simulink model "Hell_ix_System_Architecture"  (R2022b)
settings: Solver=VariableStepAuto  StartTime=0.0  StopTime=10.0  RelTol=1e-3
(part 1 of 2)
settings Model: Creator=Daniel Sotelo  LastModifiedBy=Daniel Sotelo

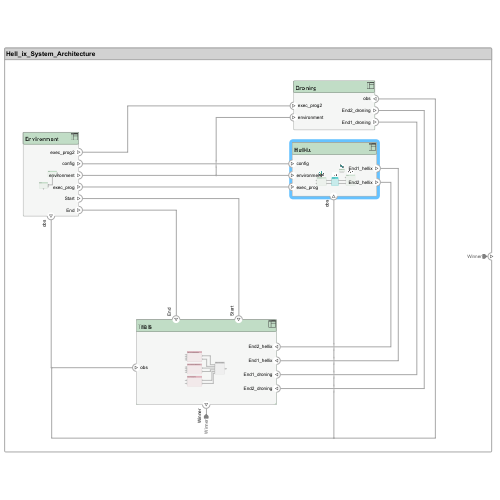
[thumbnail: Simulink's stored preview of the top-level diagram]
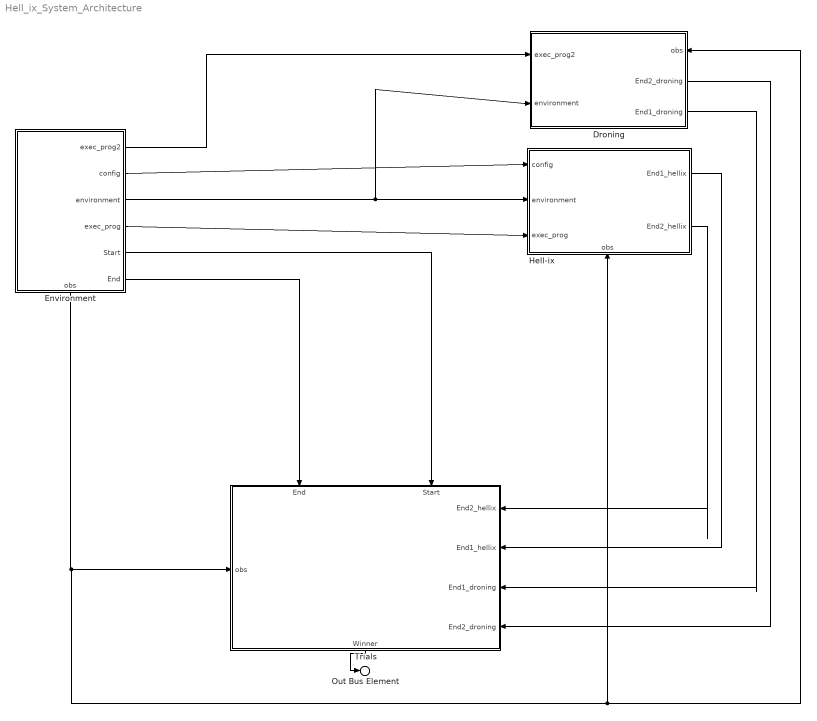
== system Hell_ix_System_Architecture ==
  Droning : Subsystem
      settings: PortSchema="{\"entries\":[{\"content\":{\"headerSize\":26,\"margin\":15,\"minimumSpacing\":25,\"sides\":[{\"content\":{\"connectorIds\":[\"In2\",\"In1\"]},\"type\":\"ConnectorPlacement.EquallySpacedRectSide\",\"uuid\":\"e97e1fd1-9f1b-43cc-bf15-a23fe97b9f57\"},{\"content\":{\"connectorIds\":[\"In3\",\"Out2\",\"Out1\"],\"side\":\"RIGHT\"},\"type\":\"ConnectorPlacement.EquallySpacedRectSide\",\"uuid\":\"b384b9c5-fcee-4054-b020-18cc4d409726\"},{\"content\":{\"connectorIds\":[],\"side\":\"TOP\"},\"type\":\"ConnectorPlacement.EquallySpacedRectSide\",\"uuid\":\"0ff74274-cc13-4bc9-ab97-befa0144ddb0\"}]},\"type\":\"ConnectorPlacement.EquallySpacedConnector\",\"uuid\":\"32a64cae-dc0e-47e5-be72-f6041fa7e3a1\"}],\"packageUris\":[\"http://schema.mathworks.com/mf0/Connector/R2020b\"],\"version\":\"1.0\"}"
  Environment : Subsystem
      settings: PortSchema="{\"entries\":[{\"content\":{\"headerSize\":26,\"margin\":15,\"minimumSpacing\":25,\"sides\":[{\"content\":{\"connectorIds\":[]},\"type\":\"ConnectorPlacement.EquallySpacedRectSide\",\"uuid\":\"e97e1fd1-9f1b-43cc-bf15-a23fe97b9f57\"},{\"content\":{\"connectorIds\":[\"Out3\",\"Out2\",\"Out1\",\"Out4\",\"Out5\",\"Out6\"],\"side\":\"RIGHT\"},\"type\":\"ConnectorPlacement.EquallySpacedRectSide\",\"uuid\":\"b384b9c5-fcee-4054-b020-18cc4d409726\"},{\"content\":{\"connectorIds\":[],\"side\":\"TOP\"},\"type\":\"ConnectorPlacement.EquallySpacedRectSide\",\"uuid\":\"0ff74274-cc13-4bc9-ab97-befa0144ddb0\"},{\"content\":{\"connectorIds\":[\"Out7\"],\"side\":\"BOTTOM\"},\"type\":\"ConnectorPlacement.EquallySpacedRectSide\",\"uuid\":\"34d21596-7255-4b53-b653-035a383f4a5b\"}]},\"type\":\"ConnectorPlacement.EquallySpacedConnector\",\"uuid\":\"32a64cae-dc0e-47e5-be72-f6041fa7e3a1\"}],\"packageUris\":[\"http://schema.mathworks.com/mf0/Connector/R2020b\"],\"version\":\"1.0\"}"
  Hell-ix : Subsystem
      settings: PortSchema="{\"entries\":[{\"content\":{\"headerSize\":26,\"margin\":15,\"minimumSpacing\":25,\"sides\":[{\"content\":{\"connectorIds\":[\"In1\",\"In2\",\"In3\"]},\"type\":\"ConnectorPlacement.EquallySpacedRectSide\",\"uuid\":\"e97e1fd1-9f1b-43cc-bf15-a23fe97b9f57\"},{\"content\":{\"connectorIds\":[\"Out2\",\"Out1\"],\"side\":\"RIGHT\"},\"type\":\"ConnectorPlacement.EquallySpacedRectSide\",\"uuid\":\"b384b9c5-fcee-4054-b020-18cc4d409726\"},{\"content\":{\"connectorIds\":[],\"side\":\"TOP\"},\"type\":\"ConnectorPlacement.EquallySpacedRectSide\",\"uuid\":\"0ff74274-cc13-4bc9-ab97-befa0144ddb0\"},{\"content\":{\"connectorIds\":[\"In4\"],\"side\":\"BOTTOM\"},\"type\":\"ConnectorPlacement.EquallySpacedRectSide\",\"uuid\":\"8630347b-1320-4b67-a4d6-78d4ff5f81b4\"}]},\"type\":\"ConnectorPlacement.EquallySpacedConnector\",\"uuid\":\"32a64cae-dc0e-47e5-be72-f6041fa7e3a1\"}],\"packageUris\":[\"http://schema.mathworks.com/mf0/Connector/R2020b\"],\"version\":\"1.0\"}"
  Trials : Subsystem
      settings: PortSchema="{\"entries\":[{\"content\":{\"headerSize\":26,\"margin\":15,\"minimumSpacing\":25,\"sides\":[{\"content\":{\"connectorIds\":[\"In7\"]},\"type\":\"ConnectorPlacement.EquallySpacedRectSide\",\"uuid\":\"e97e1fd1-9f1b-43cc-bf15-a23fe97b9f57\"},{\"content\":{\"connectorIds\":[\"In5\",\"In6\",\"In3\",\"In4\"],\"side\":\"RIGHT\"},\"type\":\"ConnectorPlacement.EquallySpacedRectSide\",\"uuid\":\"b384b9c5-fcee-4054-b020-18cc4d409726\"},{\"content\":{\"connectorIds\":[\"In2\",\"In1\"],\"side\":\"TOP\"},\"type\":\"ConnectorPlacement.EquallySpacedRectSide\",\"uuid\":\"0ff74274-cc13-4bc9-ab97-befa0144ddb0\"},{\"content\":{\"connectorIds\":[\"Out1\"],\"side\":\"BOTTOM\"},\"type\":\"ConnectorPlacement.EquallySpacedRectSide\",\"uuid\":\"9cacfc43-c38e-4776-99af-1c6d2f7a9023\"}]},\"type\":\"ConnectorPlacement.EquallySpacedConnector\",\"uuid\":\"32a64cae-dc0e-47e5-be72-f6041fa7e3a1\"}],\"packageUris\":[\"http://schema.mathworks.com/mf0/Connector/R2020b\"],\"version\":\"1.0\"}"
  Out Bus Element : Outport  PortName=Winner
  wires:
  Environment/4(exec_prog) -> Hell-ix/3(exec_prog)
  Environment/7(obs) -> Trials/7(obs), Hell-ix/4(obs), Droning/3(obs)
  Environment/6(End) -> Trials/2(End)
  Environment/3(exec_prog2) -> Droning/2(exec_prog2)
  Environment/5(Start) -> Trials/1(Start)
  Environment/1(environment) -> Droning/1(environment), Hell-ix/2(environment)
  Droning/1(End1_droning) -> Trials/3(End1_droning)
  Droning/2(End2_droning) -> Trials/4(End2_droning)
  Hell-ix/1(End2_hellix) -> Trials/5(End2_hellix)
  Hell-ix/2(End1_hellix) -> Trials/6(End1_hellix)
  Trials/1(Winner) -> Out Bus Element/1
  Environment/2(config) -> Hell-ix/1(config)

== system Hell_ix_System_Architecture/Droning ==
  Bus Element In3 : Inport  PortName=environment
  Bus Element In1 : Inport  Port=2  PortName=exec_prog2
  Bus Element In2 : Inport  Port=3  PortName=obs
  Bus Element Out1 : Outport  PortName=End1_droning
  Bus Element Out2 : Outport  Port=2  PortName=End2_droning

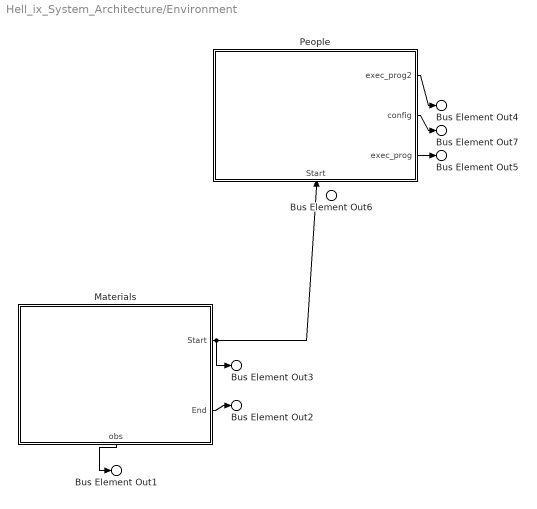
== system Hell_ix_System_Architecture/Environment ==
  Materials : Subsystem
      settings: PortSchema="{\"entries\":[{\"content\":{\"headerSize\":26,\"margin\":15,\"minimumSpacing\":25,\"sides\":[{\"content\":{\"connectorIds\":[]},\"type\":\"ConnectorPlacement.EquallySpacedRectSide\",\"uuid\":\"e97e1fd1-9f1b-43cc-bf15-a23fe97b9f57\"},{\"content\":{\"connectorIds\":[\"Out1\",\"Out3\"],\"side\":\"RIGHT\"},\"type\":\"ConnectorPlacement.EquallySpacedRectSide\",\"uuid\":\"b384b9c5-fcee-4054-b020-18cc4d409726\"},{\"content\":{\"connectorIds\":[],\"side\":\"TOP\"},\"type\":\"ConnectorPlacement.EquallySpacedRectSide\",\"uuid\":\"0ff74274-cc13-4bc9-ab97-befa0144ddb0\"},{\"content\":{\"connectorIds\":[\"Out2\"],\"side\":\"BOTTOM\"},\"type\":\"ConnectorPlacement.EquallySpacedRectSide\",\"uuid\":\"156d3aac-f76d-47d1-8807-e77bc3f5e7ef\"}]},\"type\":\"ConnectorPlacement.EquallySpacedConnector\",\"uuid\":\"32a64cae-dc0e-47e5-be72-f6041fa7e3a1\"}],\"packageUris\":[\"http://schema.mathworks.com/mf0/Connector/R2020b\"],\"version\":\"1.0\"}"
  People : Subsystem
      settings: PortSchema="{\"entries\":[{\"content\":{\"headerSize\":26,\"margin\":15,\"minimumSpacing\":25,\"sides\":[{\"content\":{\"connectorIds\":[]},\"type\":\"ConnectorPlacement.EquallySpacedRectSide\",\"uuid\":\"e97e1fd1-9f1b-43cc-bf15-a23fe97b9f57\"},{\"content\":{\"connectorIds\":[\"Out3\",\"Out2\",\"Out1\"],\"side\":\"RIGHT\"},\"type\":\"ConnectorPlacement.EquallySpacedRectSide\",\"uuid\":\"b384b9c5-fcee-4054-b020-18cc4d409726\"},{\"content\":{\"connectorIds\":[],\"side\":\"TOP\"},\"type\":\"ConnectorPlacement.EquallySpacedRectSide\",\"uuid\":\"0ff74274-cc13-4bc9-ab97-befa0144ddb0\"},{\"content\":{\"connectorIds\":[\"In1\"],\"side\":\"BOTTOM\"},\"type\":\"ConnectorPlacement.EquallySpacedRectSide\",\"uuid\":\"a378ab0b-ffdd-4b76-9379-7a6c14cd9027\"}]},\"type\":\"ConnectorPlacement.EquallySpacedConnector\",\"uuid\":\"32a64cae-dc0e-47e5-be72-f6041fa7e3a1\"}],\"packageUris\":[\"http://schema.mathworks.com/mf0/Connector/R2020b\"],\"version\":\"1.0\"}"
  Bus Element Out6 : Outport  PortName=environment
  Bus Element Out7 : Outport  Port=2  PortName=config
  Bus Element Out4 : Outport  Port=3  PortName=exec_prog2
  Bus Element Out5 : Outport  Port=4  PortName=exec_prog
  Bus Element Out3 : Outport  Port=5  PortName=Start
  Bus Element Out2 : Outport  Port=6  PortName=End
  Bus Element Out1 : Outport  Port=7  PortName=obs
  wires:
  Materials/2(obs) -> Bus Element Out1/1
  Materials/3(End) -> Bus Element Out2/1
  Materials/1(Start) -> People/1(Start), Bus Element Out3/1
  People/3(exec_prog2) -> Bus Element Out4/1
  People/1(exec_prog) -> Bus Element Out5/1
  People/2(config) -> Bus Element Out7/1

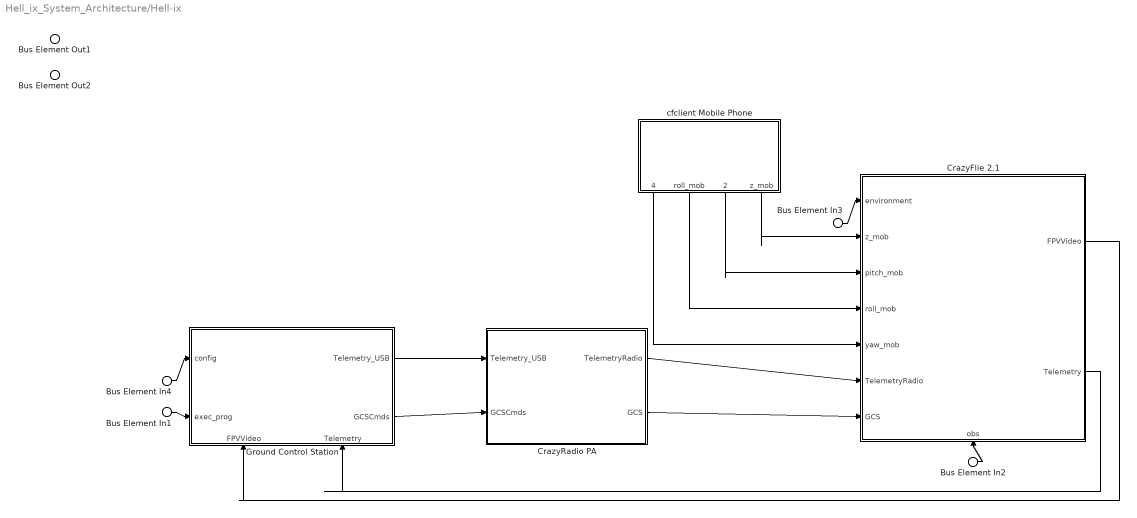
== system Hell_ix_System_Architecture/Hell-ix ==
  Bus Element In4 : Inport  PortName=config
  Bus Element In3 : Inport  Port=2  PortName=environment
  Bus Element In1 : Inport  Port=3  PortName=exec_prog
  Bus Element In2 : Inport  Port=4  PortName=obs
  CrazyFlie 2.1 : Subsystem
      settings: PortSchema="{\"entries\":[{\"content\":{\"headerSize\":26,\"margin\":15,\"minimumSpacing\":25,\"sides\":[{\"content\":{\"connectorIds\":[\"In2\",\"In4\",\"In5\",\"In6\",\"In7\",\"In3\",\"In8\"]},\"type\":\"ConnectorPlacement.EquallySpacedRectSide\",\"uuid\":\"e97e1fd1-9f1b-43cc-bf15-a23fe97b9f57\"},{\"content\":{\"connectorIds\":[\"Out2\",\"Out1\"],\"side\":\"RIGHT\"},\"type\":\"ConnectorPlacement.EquallySpacedRectSide\",\"uuid\":\"b384b9c5-fcee-4054-b020-18cc4d409726\"},{\"content\":{\"connectorIds\":[],\"side\":\"TOP\"},\"type\":\"ConnectorPlacement.EquallySpacedRectSide\",\"uuid\":\"0ff74274-cc13-4bc9-ab97-befa0144ddb0\"},{\"content\":{\"connectorIds\":[\"In1\"],\"side\":\"BOTTOM\"},\"type\":\"ConnectorPlacement.EquallySpacedRectSide\",\"uuid\":\"e7cf066c-a9d0-4f44-9f2b-ff8a675b3a93\"}]},\"type\":\"ConnectorPlacement.EquallySpacedConnector\",\"uuid\":\"32a64cae-dc0e-47e5-be72-f6041fa7e3a1\"}],\"packageUris\":[\"http://schema.mathworks.com/mf0/Connector/R2020b\"],\"version\":\"1.0\"}"
  CrazyRadio PA : Subsystem
      settings: PortSchema="{\"entries\":[{\"content\":{\"headerSize\":26,\"margin\":15,\"minimumSpacing\":25,\"sides\":[{\"content\":{\"connectorIds\":[\"In1\",\"In2\"]},\"type\":\"ConnectorPlacement.EquallySpacedRectSide\",\"uuid\":\"e97e1fd1-9f1b-43cc-bf15-a23fe97b9f57\"},{\"content\":{\"connectorIds\":[\"Out1\",\"Out2\"],\"side\":\"RIGHT\"},\"type\":\"ConnectorPlacement.EquallySpacedRectSide\",\"uuid\":\"b384b9c5-fcee-4054-b020-18cc4d409726\"},{\"content\":{\"connectorIds\":[],\"side\":\"TOP\"},\"type\":\"ConnectorPlacement.EquallySpacedRectSide\",\"uuid\":\"0ff74274-cc13-4bc9-ab97-befa0144ddb0\"}]},\"type\":\"ConnectorPlacement.EquallySpacedConnector\",\"uuid\":\"32a64cae-dc0e-47e5-be72-f6041fa7e3a1\"}],\"packageUris\":[\"http://schema.mathworks.com/mf0/Connector/R2020b\"],\"version\":\"1.0\"}"
  Ground Control Station : Subsystem
      settings: PortSchema="{\"entries\":[{\"content\":{\"headerSize\":26,\"margin\":15,\"minimumSpacing\":25,\"sides\":[{\"content\":{\"connectorIds\":[\"In1\",\"In2\"]},\"type\":\"ConnectorPlacement.EquallySpacedRectSide\",\"uuid\":\"e97e1fd1-9f1b-43cc-bf15-a23fe97b9f57\"},{\"content\":{\"connectorIds\":[\"Out1\",\"Out2\"],\"side\":\"RIGHT\"},\"type\":\"ConnectorPlacement.EquallySpacedRectSide\",\"uuid\":\"b384b9c5-fcee-4054-b020-18cc4d409726\"},{\"content\":{\"connectorIds\":[],\"side\":\"TOP\"},\"type\":\"ConnectorPlacement.EquallySpacedRectSide\",\"uuid\":\"0ff74274-cc13-4bc9-ab97-befa0144ddb0\"},{\"content\":{\"connectorIds\":[\"In3\",\"In4\"],\"side\":\"BOTTOM\"},\"type\":\"ConnectorPlacement.EquallySpacedRectSide\",\"uuid\":\"d255ce1e-bd8c-464a-9c5c-901bed1a1a29\"}]},\"type\":\"ConnectorPlacement.EquallySpacedConnector\",\"uuid\":\"32a64cae-dc0e-47e5-be72-f6041fa7e3a1\"}],\"packageUris\":[\"http://schema.mathworks.com/mf0/Connector/R2020b\"],\"version\":\"1.0\"}"
  cfclient Mobile Phone : Subsystem
      settings: PortSchema="{\"entries\":[{\"content\":{\"headerSize\":26,\"margin\":15,\"minimumSpacing\":25,\"sides\":[{\"content\":{\"connectorIds\":[]},\"type\":\"ConnectorPlacement.EquallySpacedRectSide\",\"uuid\":\"e97e1fd1-9f1b-43cc-bf15-a23fe97b9f57\"},{\"content\":{\"connectorIds\":[],\"side\":\"RIGHT\"},\"type\":\"ConnectorPlacement.EquallySpacedRectSide\",\"uuid\":\"b384b9c5-fcee-4054-b020-18cc4d409726\"},{\"content\":{\"connectorIds\":[],\"side\":\"TOP\"},\"type\":\"ConnectorPlacement.EquallySpacedRectSide\",\"uuid\":\"0ff74274-cc13-4bc9-ab97-befa0144ddb0\"},{\"content\":{\"connectorIds\":[\"Out4\",\"Out3\",\"Out2\",\"Out1\"],\"side\":\"BOTTOM\"},\"type\":\"ConnectorPlacement.EquallySpacedRectSide\",\"uuid\":\"6bcd37d7-be34-4491-8512-8c3ebf2e5fa9\"}]},\"type\":\"ConnectorPlacement.EquallySpacedConnector\",\"uuid\":\"32a64cae-dc0e-47e5-be72-f6041fa7e3a1\"}],\"packageUris\":[\"http://schema.mathworks.com/mf0/Connector/R2020b\"],\"version\":\"1.0\"}"
  Bus Element Out1 : Outport  PortName=End2_hellix
  Bus Element Out2 : Outport  Port=2  PortName=End1_hellix
  wires:
  Ground Control Station/1(Telemetry_USB) -> CrazyRadio PA/1(Telemetry_USB)
  Ground Control Station/2(GCSCmds) -> CrazyRadio PA/2(GCSCmds)
  CrazyRadio PA/2(GCS) -> CrazyFlie 2.1/8(GCS)
  CrazyRadio PA/1(TelemetryRadio) -> CrazyFlie 2.1/3(TelemetryRadio)
  Bus Element In1/1 -> Ground Control Station/2(exec_prog)
  Bus Element In4/1 -> Ground Control Station/1(config)
  Bus Element In3/1 -> CrazyFlie 2.1/2(environment)
  CrazyFlie 2.1/2(FPVVideo) -> Ground Control Station/3(FPVVideo)
  cfclient Mobile Phone/1(z_mob) -> CrazyFlie 2.1/4(z_mob)
  cfclient Mobile Phone/2(pitch_mob) -> CrazyFlie 2.1/5(pitch_mob)
  cfclient Mobile Phone/3(roll_mob) -> CrazyFlie 2.1/6(roll_mob)
  cfclient Mobile Phone/4(yaw_mob) -> CrazyFlie 2.1/7(yaw_mob)
  Bus Element In2/1 -> CrazyFlie 2.1/1(obs)
  CrazyFlie 2.1/1(Telemetry) -> Ground Control Station/4(Telemetry)

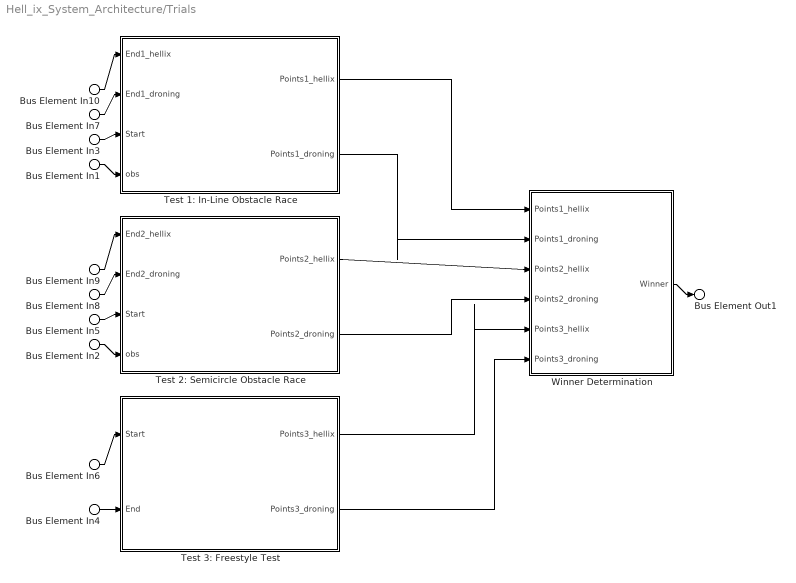
== system Hell_ix_System_Architecture/Trials ==
  Bus Element In3 : Inport  PortName=Start
  Bus Element In5 : Inport  PortName=Start
  Bus Element In6 : Inport  PortName=Start
  Bus Element In4 : Inport  Port=2  PortName=End
  Bus Element In7 : Inport  Port=3  PortName=End1_droning
  Bus Element In8 : Inport  Port=4  PortName=End2_droning
  Bus Element In9 : Inport  Port=5  PortName=End2_hellix
  Bus Element In10 : Inport  Port=6  PortName=End1_hellix
  Bus Element In1 : Inport  Port=7  PortName=obs
  Bus Element In2 : Inport  Port=7  PortName=obs
  Test 1: In-Line Obstacle Race : Subsystem
      settings: PortSchema="{\"entries\":[{\"content\":{\"headerSize\":26,\"margin\":15,\"minimumSpacing\":25,\"sides\":[{\"content\":{\"connectorIds\":[\"In1\",\"In2\",\"In3\",\"In4\"]},\"type\":\"ConnectorPlacement.EquallySpacedRectSide\",\"uuid\":\"e97e1fd1-9f1b-43cc-bf15-a23fe97b9f57\"},{\"content\":{\"connectorIds\":[\"Out1\",\"Out2\"],\"side\":\"RIGHT\"},\"type\":\"ConnectorPlacement.EquallySpacedRectSide\",\"uuid\":\"b384b9c5-fcee-4054-b020-18cc4d409726\"},{\"content\":{\"connectorIds\":[],\"side\":\"TOP\"},\"type\":\"ConnectorPlacement.EquallySpacedRectSide\",\"uuid\":\"0ff74274-cc13-4bc9-ab97-befa0144ddb0\"}]},\"type\":\"ConnectorPlacement.EquallySpacedConnector\",\"uuid\":\"32a64cae-dc0e-47e5-be72-f6041fa7e3a1\"}],\"packageUris\":[\"http://schema.mathworks.com/mf0/Connector/R2020b\"],\"version\":\"1.0\"}"
  Test 2: Semicircle Obstacle Race : Subsystem
      settings: PortSchema="{\"entries\":[{\"content\":{\"headerSize\":26,\"margin\":15,\"minimumSpacing\":25,\"sides\":[{\"content\":{\"connectorIds\":[\"In1\",\"In2\",\"In3\",\"In4\"]},\"type\":\"ConnectorPlacement.EquallySpacedRectSide\",\"uuid\":\"e97e1fd1-9f1b-43cc-bf15-a23fe97b9f57\"},{\"content\":{\"connectorIds\":[\"Out1\",\"Out2\"],\"side\":\"RIGHT\"},\"type\":\"ConnectorPlacement.EquallySpacedRectSide\",\"uuid\":\"b384b9c5-fcee-4054-b020-18cc4d409726\"},{\"content\":{\"connectorIds\":[],\"side\":\"TOP\"},\"type\":\"ConnectorPlacement.EquallySpacedRectSide\",\"uuid\":\"0ff74274-cc13-4bc9-ab97-befa0144ddb0\"}]},\"type\":\"ConnectorPlacement.EquallySpacedConnector\",\"uuid\":\"32a64cae-dc0e-47e5-be72-f6041fa7e3a1\"}],\"packageUris\":[\"http://schema.mathworks.com/mf0/Connector/R2020b\"],\"version\":\"1.0\"}"
  Test 3: Freestyle Test : Subsystem
      settings: PortSchema="{\"entries\":[{\"content\":{\"headerSize\":26,\"margin\":15,\"minimumSpacing\":25,\"sides\":[{\"content\":{\"connectorIds\":[\"In1\",\"In2\"]},\"type\":\"ConnectorPlacement.EquallySpacedRectSide\",\"uuid\":\"e97e1fd1-9f1b-43cc-bf15-a23fe97b9f57\"},{\"content\":{\"connectorIds\":[\"Out1\",\"Out2\"],\"side\":\"RIGHT\"},\"type\":\"ConnectorPlacement.EquallySpacedRectSide\",\"uuid\":\"b384b9c5-fcee-4054-b020-18cc4d409726\"},{\"content\":{\"connectorIds\":[],\"side\":\"TOP\"},\"type\":\"ConnectorPlacement.EquallySpacedRectSide\",\"uuid\":\"0ff74274-cc13-4bc9-ab97-befa0144ddb0\"}]},\"type\":\"ConnectorPlacement.EquallySpacedConnector\",\"uuid\":\"32a64cae-dc0e-47e5-be72-f6041fa7e3a1\"}],\"packageUris\":[\"http://schema.mathworks.com/mf0/Connector/R2020b\"],\"version\":\"1.0\"}"
  Winner Determination : Subsystem
      settings: PortSchema="{\"entries\":[{\"content\":{\"headerSize\":26,\"margin\":15,\"minimumSpacing\":25,\"sides\":[{\"content\":{\"connectorIds\":[\"In2\",\"In1\",\"In3\",\"In4\",\"In6\",\"In5\"]},\"type\":\"ConnectorPlacement.EquallySpacedRectSide\",\"uuid\":\"e97e1fd1-9f1b-43cc-bf15-a23fe97b9f57\"},{\"content\":{\"connectorIds\":[\"Out1\"],\"side\":\"RIGHT\"},\"type\":\"ConnectorPlacement.EquallySpacedRectSide\",\"uuid\":\"b384b9c5-fcee-4054-b020-18cc4d409726\"},{\"content\":{\"connectorIds\":[],\"side\":\"TOP\"},\"type\":\"ConnectorPlacement.EquallySpacedRectSide\",\"uuid\":\"0ff74274-cc13-4bc9-ab97-befa0144ddb0\"}]},\"type\":\"ConnectorPlacement.EquallySpacedConnector\",\"uuid\":\"32a64cae-dc0e-47e5-be72-f6041fa7e3a1\"}],\"packageUris\":[\"http://schema.mathworks.com/mf0/Connector/R2020b\"],\"version\":\"1.0\"}"
  Bus Element Out1 : Outport  PortName=Winner
  wires:
  Bus Element In1/1 -> Test 1: In-Line Obstacle Race/4(obs)
  Bus Element In2/1 -> Test 2: Semicircle Obstacle Race/4(obs)
  Bus Element In3/1 -> Test 1: In-Line Obstacle Race/3(Start)
  Bus Element In5/1 -> Test 2: Semicircle Obstacle Race/3(Start)
  Bus Element In6/1 -> Test 3: Freestyle Test/1(Start)
  Bus Element In4/1 -> Test 3: Freestyle Test/2(End)
  Bus Element In7/1 -> Test 1: In-Line Obstacle Race/2(End1_droning)
  Bus Element In10/1 -> Test 1: In-Line Obstacle Race/1(End1_hellix)
  Bus Element In8/1 -> Test 2: Semicircle Obstacle Race/2(End2_droning)
  Bus Element In9/1 -> Test 2: Semicircle Obstacle Race/1(End2_hellix)
  Test 1: In-Line Obstacle Race/1(Points1_hellix) -> Winner Determination/2(Points1_hellix)
  Test 1: In-Line Obstacle Race/2(Points1_droning) -> Winner Determination/1(Points1_droning)
  Test 2: Semicircle Obstacle Race/1(Points2_hellix) -> Winner Determination/3(Points2_hellix)
  Test 2: Semicircle Obstacle Race/2(Points2_droning) -> Winner Determination/4(Points2_droning)
  Test 3: Freestyle Test/1(Points3_hellix) -> Winner Determination/6(Points3_hellix)
  Test 3: Freestyle Test/2(Points3_droning) -> Winner Determination/5(Points3_droning)
  Winner Determination/1(Winner) -> Bus Element Out1/1

== system Hell_ix_System_Architecture/Environment/Materials ==
  Chronometer : Subsystem
      settings: PortSchema="{\"entries\":[{\"content\":{\"headerSize\":26,\"margin\":15,\"minimumSpacing\":25,\"sides\":[{\"content\":{\"connectorIds\":[\"In1\"]},\"type\":\"ConnectorPlacement.EquallySpacedRectSide\",\"uuid\":\"e97e1fd1-9f1b-43cc-bf15-a23fe97b9f57\"},{\"content\":{\"connectorIds\":[\"Out1\"],\"side\":\"RIGHT\"},\"type\":\"ConnectorPlacement.EquallySpacedRectSide\",\"uuid\":\"b384b9c5-fcee-4054-b020-18cc4d409726\"},{\"content\":{\"connectorIds\":[],\"side\":\"TOP\"},\"type\":\"ConnectorPlacement.EquallySpacedRectSide\",\"uuid\":\"0ff74274-cc13-4bc9-ab97-befa0144ddb0\"}]},\"type\":\"ConnectorPlacement.EquallySpacedConnector\",\"uuid\":\"32a64cae-dc0e-47e5-be72-f6041fa7e3a1\"}],\"packageUris\":[\"http://schema.mathworks.com/mf0/Connector/R2020b\"],\"version\":\"1.0\"}"
  Horn : Subsystem
      settings: PortSchema="{\"entries\":[{\"content\":{\"headerSize\":26,\"margin\":15,\"minimumSpacing\":25,\"sides\":[{\"content\":{\"connectorIds\":[]},\"type\":\"ConnectorPlacement.EquallySpacedRectSide\",\"uuid\":\"e97e1fd1-9f1b-43cc-bf15-a23fe97b9f57\"},{\"content\":{\"connectorIds\":[\"Out1\"],\"side\":\"RIGHT\"},\"type\":\"ConnectorPlacement.EquallySpacedRectSide\",\"uuid\":\"b384b9c5-fcee-4054-b020-18cc4d409726\"},{\"content\":{\"connectorIds\":[],\"side\":\"TOP\"},\"type\":\"ConnectorPlacement.EquallySpacedRectSide\",\"uuid\":\"0ff74274-cc13-4bc9-ab97-befa0144ddb0\"}]},\"type\":\"ConnectorPlacement.EquallySpacedConnector\",\"uuid\":\"32a64cae-dc0e-47e5-be72-f6041fa7e3a1\"}],\"packageUris\":[\"http://schema.mathworks.com/mf0/Connector/R2020b\"],\"version\":\"1.0\"}"
  Obstacles : Subsystem
      settings: PortSchema="{\"entries\":[{\"content\":{\"headerSize\":26,\"margin\":15,\"minimumSpacing\":25,\"sides\":[{\"content\":{\"connectorIds\":[]},\"type\":\"ConnectorPlacement.EquallySpacedRectSide\",\"uuid\":\"e97e1fd1-9f1b-43cc-bf15-a23fe97b9f57\"},{\"content\":{\"connectorIds\":[\"Out1\"],\"side\":\"RIGHT\"},\"type\":\"ConnectorPlacement.EquallySpacedRectSide\",\"uuid\":\"b384b9c5-fcee-4054-b020-18cc4d409726\"},{\"content\":{\"connectorIds\":[],\"side\":\"TOP\"},\"type\":\"ConnectorPlacement.EquallySpacedRectSide\",\"uuid\":\"0ff74274-cc13-4bc9-ab97-befa0144ddb0\"}]},\"type\":\"ConnectorPlacement.EquallySpacedConnector\",\"uuid\":\"32a64cae-dc0e-47e5-be72-f6041fa7e3a1\"}],\"packageUris\":[\"http://schema.mathworks.com/mf0/Connector/R2020b\"],\"version\":\"1.0\"}"
  Recording Cameras : Subsystem
      settings: PortSchema="{\"entries\":[{\"content\":{\"headerSize\":26,\"margin\":15,\"minimumSpacing\":25,\"sides\":[{\"content\":{\"connectorIds\":[\"In1\"]},\"type\":\"ConnectorPlacement.EquallySpacedRectSide\",\"uuid\":\"e97e1fd1-9f1b-43cc-bf15-a23fe97b9f57\"},{\"content\":{\"connectorIds\":[\"In2\"],\"side\":\"RIGHT\"},\"type\":\"ConnectorPlacement.EquallySpacedRectSide\",\"uuid\":\"b384b9c5-fcee-4054-b020-18cc4d409726\"},{\"content\":{\"connectorIds\":[],\"side\":\"TOP\"},\"type\":\"ConnectorPlacement.EquallySpacedRectSide\",\"uuid\":\"0ff74274-cc13-4bc9-ab97-befa0144ddb0\"}]},\"type\":\"ConnectorPlacement.EquallySpacedConnector\",\"uuid\":\"32a64cae-dc0e-47e5-be72-f6041fa7e3a1\"}],\"packageUris\":[\"http://schema.mathworks.com/mf0/Connector/R2020b\"],\"version\":\"1.0\"}"
  Bus Element Out2 : Outport  PortName=Start
  Bus Element Out3 : Outport  Port=2  PortName=obs
  Bus Element Out1 : Outport  Port=3  PortName=End
  wires:
  Chronometer/1(End) -> Recording Cameras/1(End), Bus Element Out1/1
  Horn/1(Start) -> Recording Cameras/2(Start), Chronometer/1(Start), Bus Element Out2/1
  Obstacles/1(obs) -> Bus Element Out3/1

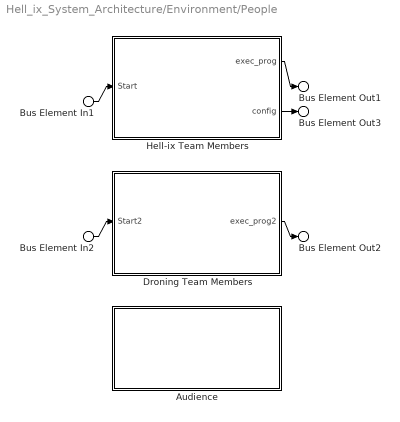
== system Hell_ix_System_Architecture/Environment/People ==
  Bus Element In1 : Inport  PortName=Start
  Bus Element In2 : Inport  PortName=Start
  Audience : Subsystem
      settings: PortSchema="{\"entries\":[{\"content\":{\"headerSize\":26,\"margin\":15,\"minimumSpacing\":25,\"sides\":[{\"content\":{\"connectorIds\":[]},\"type\":\"ConnectorPlacement.EquallySpacedRectSide\",\"uuid\":\"e97e1fd1-9f1b-43cc-bf15-a23fe97b9f57\"},{\"content\":{\"connectorIds\":[],\"side\":\"RIGHT\"},\"type\":\"ConnectorPlacement.EquallySpacedRectSide\",\"uuid\":\"b384b9c5-fcee-4054-b020-18cc4d409726\"},{\"content\":{\"connectorIds\":[],\"side\":\"TOP\"},\"type\":\"ConnectorPlacement.EquallySpacedRectSide\",\"uuid\":\"0ff74274-cc13-4bc9-ab97-befa0144ddb0\"}]},\"type\":\"ConnectorPlacement.EquallySpacedConnector\",\"uuid\":\"32a64cae-dc0e-47e5-be72-f6041fa7e3a1\"}],\"packageUris\":[\"http://schema.mathworks.com/mf0/Connector/R2020b\"],\"version\":\"1.0\"}"
  Droning Team Members : Subsystem
      settings: PortSchema="{\"entries\":[{\"content\":{\"headerSize\":26,\"margin\":15,\"minimumSpacing\":25,\"sides\":[{\"content\":{\"connectorIds\":[\"In1\"]},\"type\":\"ConnectorPlacement.EquallySpacedRectSide\",\"uuid\":\"e97e1fd1-9f1b-43cc-bf15-a23fe97b9f57\"},{\"content\":{\"connectorIds\":[\"Out1\"],\"side\":\"RIGHT\"},\"type\":\"ConnectorPlacement.EquallySpacedRectSide\",\"uuid\":\"b384b9c5-fcee-4054-b020-18cc4d409726\"},{\"content\":{\"connectorIds\":[],\"side\":\"TOP\"},\"type\":\"ConnectorPlacement.EquallySpacedRectSide\",\"uuid\":\"0ff74274-cc13-4bc9-ab97-befa0144ddb0\"}]},\"type\":\"ConnectorPlacement.EquallySpacedConnector\",\"uuid\":\"32a64cae-dc0e-47e5-be72-f6041fa7e3a1\"}],\"packageUris\":[\"http://schema.mathworks.com/mf0/Connector/R2020b\"],\"version\":\"1.0\"}"
  Hell-ix Team Members : Subsystem
      settings: PortSchema="{\"entries\":[{\"content\":{\"headerSize\":26,\"margin\":15,\"minimumSpacing\":25,\"sides\":[{\"content\":{\"connectorIds\":[\"In1\"]},\"type\":\"ConnectorPlacement.EquallySpacedRectSide\",\"uuid\":\"e97e1fd1-9f1b-43cc-bf15-a23fe97b9f57\"},{\"content\":{\"connectorIds\":[\"Out1\",\"Out2\"],\"side\":\"RIGHT\"},\"type\":\"ConnectorPlacement.EquallySpacedRectSide\",\"uuid\":\"b384b9c5-fcee-4054-b020-18cc4d409726\"},{\"content\":{\"connectorIds\":[],\"side\":\"TOP\"},\"type\":\"ConnectorPlacement.EquallySpacedRectSide\",\"uuid\":\"0ff74274-cc13-4bc9-ab97-befa0144ddb0\"}]},\"type\":\"ConnectorPlacement.EquallySpacedConnector\",\"uuid\":\"32a64cae-dc0e-47e5-be72-f6041fa7e3a1\"}],\"packageUris\":[\"http://schema.mathworks.com/mf0/Connector/R2020b\"],\"version\":\"1.0\"}"
  Bus Element Out1 : Outport  PortName=exec_prog
  Bus Element Out3 : Outport  Port=2  PortName=config
  Bus Element Out2 : Outport  Port=3  PortName=exec_prog2
  wires:
  Bus Element In1/1 -> Hell-ix Team Members/1(Start)
  Hell-ix Team Members/1(exec_prog) -> Bus Element Out1/1
  Droning Team Members/1(exec_prog2) -> Bus Element Out2/1
  Bus Element In2/1 -> Droning Team Members/1(Start2)
  Hell-ix Team Members/2(config) -> Bus Element Out3/1

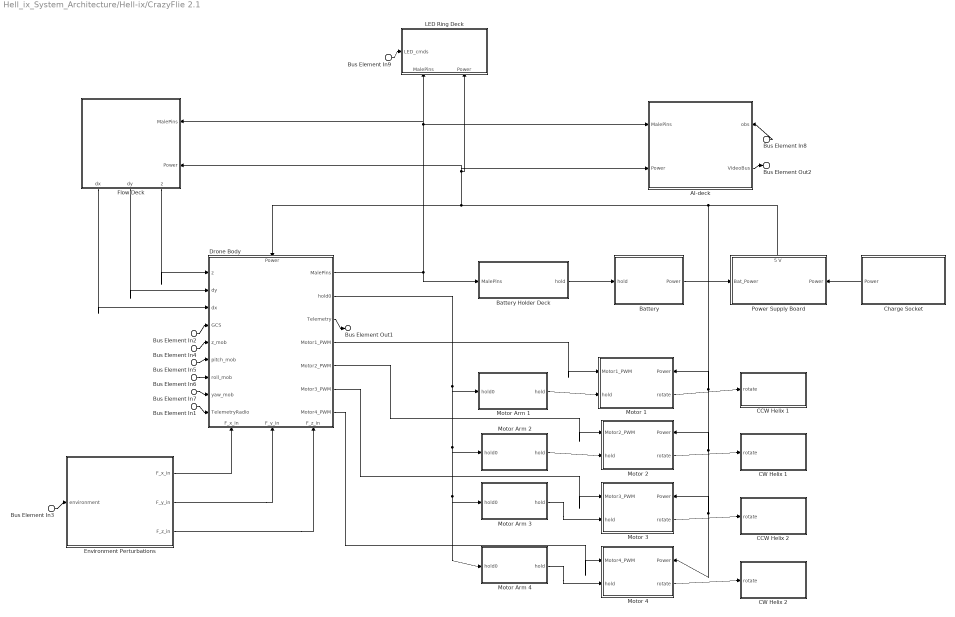
== system Hell_ix_System_Architecture/Hell-ix/CrazyFlie 2.1 ==
  Bus Element In8 : Inport  PortName=obs
  Bus Element In3 : Inport  Port=2  PortName=environment
  Bus Element In9 : Inport  Port=3  PortName=TelemetryRadio
  Bus Element In1 : Inport  Port=3  PortName=TelemetryRadio
  Bus Element In4 : Inport  Port=4  PortName=z_mob
  Bus Element In5 : Inport  Port=5  PortName=pitch_mob
  Bus Element In6 : Inport  Port=6  PortName=roll_mob
  Bus Element In7 : Inport  Port=7  PortName=yaw_mob
  Bus Element In2 : Inport  Port=8  PortName=GCS
  AI-deck : Subsystem
      settings: PortSchema="{\"entries\":[{\"content\":{\"headerSize\":26,\"margin\":15,\"minimumSpacing\":25,\"sides\":[{\"content\":{\"connectorIds\":[\"In2\",\"In3\"]},\"type\":\"ConnectorPlacement.EquallySpacedRectSide\",\"uuid\":\"e97e1fd1-9f1b-43cc-bf15-a23fe97b9f57\"},{\"content\":{\"connectorIds\":[\"In1\",\"Out1\"],\"side\":\"RIGHT\"},\"type\":\"ConnectorPlacement.EquallySpacedRectSide\",\"uuid\":\"b384b9c5-fcee-4054-b020-18cc4d409726\"},{\"content\":{\"connectorIds\":[],\"side\":\"TOP\"},\"type\":\"ConnectorPlacement.EquallySpacedRectSide\",\"uuid\":\"0ff74274-cc13-4bc9-ab97-befa0144ddb0\"}]},\"type\":\"ConnectorPlacement.EquallySpacedConnector\",\"uuid\":\"32a64cae-dc0e-47e5-be72-f6041fa7e3a1\"}],\"packageUris\":[\"http://schema.mathworks.com/mf0/Connector/R2020b\"],\"version\":\"1.0\"}"
  Battery : Subsystem
      settings: PortSchema="{\"entries\":[{\"content\":{\"headerSize\":26,\"margin\":15,\"minimumSpacing\":25,\"sides\":[{\"content\":{\"connectorIds\":[\"In1\"]},\"type\":\"ConnectorPlacement.EquallySpacedRectSide\",\"uuid\":\"e97e1fd1-9f1b-43cc-bf15-a23fe97b9f57\"},{\"content\":{\"connectorIds\":[\"Out1\"],\"side\":\"RIGHT\"},\"type\":\"ConnectorPlacement.EquallySpacedRectSide\",\"uuid\":\"b384b9c5-fcee-4054-b020-18cc4d409726\"},{\"content\":{\"connectorIds\":[],\"side\":\"TOP\"},\"type\":\"ConnectorPlacement.EquallySpacedRectSide\",\"uuid\":\"0ff74274-cc13-4bc9-ab97-befa0144ddb0\"}]},\"type\":\"ConnectorPlacement.EquallySpacedConnector\",\"uuid\":\"32a64cae-dc0e-47e5-be72-f6041fa7e3a1\"}],\"packageUris\":[\"http://schema.mathworks.com/mf0/Connector/R2020b\"],\"version\":\"1.0\"}"
  Battery Holder Deck : Subsystem
      settings: PortSchema="{\"entries\":[{\"content\":{\"headerSize\":26,\"margin\":15,\"minimumSpacing\":25,\"sides\":[{\"content\":{\"connectorIds\":[\"In1\"]},\"type\":\"ConnectorPlacement.EquallySpacedRectSide\",\"uuid\":\"e97e1fd1-9f1b-43cc-bf15-a23fe97b9f57\"},{\"content\":{\"connectorIds\":[\"Out1\"],\"side\":\"RIGHT\"},\"type\":\"ConnectorPlacement.EquallySpacedRectSide\",\"uuid\":\"b384b9c5-fcee-4054-b020-18cc4d409726\"},{\"content\":{\"connectorIds\":[],\"side\":\"TOP\"},\"type\":\"ConnectorPlacement.EquallySpacedRectSide\",\"uuid\":\"0ff74274-cc13-4bc9-ab97-befa0144ddb0\"}]},\"type\":\"ConnectorPlacement.EquallySpacedConnector\",\"uuid\":\"32a64cae-dc0e-47e5-be72-f6041fa7e3a1\"}],\"packageUris\":[\"http://schema.mathworks.com/mf0/Connector/R2020b\"],\"version\":\"1.0\"}"
  CCW Helix 1 : Subsystem
      settings: PortSchema="{\"entries\":[{\"content\":{\"headerSize\":26,\"margin\":15,\"minimumSpacing\":25,\"sides\":[{\"content\":{\"connectorIds\":[\"In1\"]},\"type\":\"ConnectorPlacement.EquallySpacedRectSide\",\"uuid\":\"e97e1fd1-9f1b-43cc-bf15-a23fe97b9f57\"},{\"content\":{\"connectorIds\":[],\"side\":\"RIGHT\"},\"type\":\"ConnectorPlacement.EquallySpacedRectSide\",\"uuid\":\"b384b9c5-fcee-4054-b020-18cc4d409726\"},{\"content\":{\"connectorIds\":[],\"side\":\"TOP\"},\"type\":\"ConnectorPlacement.EquallySpacedRectSide\",\"uuid\":\"0ff74274-cc13-4bc9-ab97-befa0144ddb0\"},{\"content\":{\"connectorIds\":[],\"side\":\"BOTTOM\"},\"type\":\"ConnectorPlacement.EquallySpacedRectSide\",\"uuid\":\"b4539d99-d74c-48ec-aeba-e1211e6ae847\"}]},\"type\":\"ConnectorPlacement.EquallySpacedConnector\",\"uuid\":\"32a64cae-dc0e-47e5-be72-f6041fa7e3a1\"}],\"packageUris\":[\"http://schema.mathworks.com/mf0/Connector/R2020b\"],\"version\":\"1.0\"}"
  CCW Helix 2 : Subsystem
      settings: PortSchema="{\"entries\":[{\"content\":{\"headerSize\":26,\"margin\":15,\"minimumSpacing\":25,\"sides\":[{\"content\":{\"connectorIds\":[\"In1\"]},\"type\":\"ConnectorPlacement.EquallySpacedRectSide\",\"uuid\":\"e97e1fd1-9f1b-43cc-bf15-a23fe97b9f57\"},{\"content\":{\"connectorIds\":[],\"side\":\"RIGHT\"},\"type\":\"ConnectorPlacement.EquallySpacedRectSide\",\"uuid\":\"b384b9c5-fcee-4054-b020-18cc4d409726\"},{\"content\":{\"connectorIds\":[],\"side\":\"TOP\"},\"type\":\"ConnectorPlacement.EquallySpacedRectSide\",\"uuid\":\"0ff74274-cc13-4bc9-ab97-befa0144ddb0\"},{\"content\":{\"connectorIds\":[],\"side\":\"BOTTOM\"},\"type\":\"ConnectorPlacement.EquallySpacedRectSide\",\"uuid\":\"b4539d99-d74c-48ec-aeba-e1211e6ae847\"}]},\"type\":\"ConnectorPlacement.EquallySpacedConnector\",\"uuid\":\"32a64cae-dc0e-47e5-be72-f6041fa7e3a1\"}],\"packageUris\":[\"http://schema.mathworks.com/mf0/Connector/R2020b\"],\"version\":\"1.0\"}"
  CW Helix 1 : Subsystem
      settings: PortSchema="{\"entries\":[{\"content\":{\"headerSize\":26,\"margin\":15,\"minimumSpacing\":25,\"sides\":[{\"content\":{\"connectorIds\":[\"In1\"]},\"type\":\"ConnectorPlacement.EquallySpacedRectSide\",\"uuid\":\"e97e1fd1-9f1b-43cc-bf15-a23fe97b9f57\"},{\"content\":{\"connectorIds\":[],\"side\":\"RIGHT\"},\"type\":\"ConnectorPlacement.EquallySpacedRectSide\",\"uuid\":\"b384b9c5-fcee-4054-b020-18cc4d409726\"},{\"content\":{\"connectorIds\":[],\"side\":\"TOP\"},\"type\":\"ConnectorPlacement.EquallySpacedRectSide\",\"uuid\":\"0ff74274-cc13-4bc9-ab97-befa0144ddb0\"},{\"content\":{\"connectorIds\":[],\"side\":\"BOTTOM\"},\"type\":\"ConnectorPlacement.EquallySpacedRectSide\",\"uuid\":\"b4539d99-d74c-48ec-aeba-e1211e6ae847\"}]},\"type\":\"ConnectorPlacement.EquallySpacedConnector\",\"uuid\":\"32a64cae-dc0e-47e5-be72-f6041fa7e3a1\"}],\"packageUris\":[\"http://schema.mathworks.com/mf0/Connector/R2020b\"],\"version\":\"1.0\"}"
  CW Helix 2 : Subsystem
      settings: PortSchema="{\"entries\":[{\"content\":{\"headerSize\":26,\"margin\":15,\"minimumSpacing\":25,\"sides\":[{\"content\":{\"connectorIds\":[\"In1\"]},\"type\":\"ConnectorPlacement.EquallySpacedRectSide\",\"uuid\":\"e97e1fd1-9f1b-43cc-bf15-a23fe97b9f57\"},{\"content\":{\"connectorIds\":[],\"side\":\"RIGHT\"},\"type\":\"ConnectorPlacement.EquallySpacedRectSide\",\"uuid\":\"b384b9c5-fcee-4054-b020-18cc4d409726\"},{\"content\":{\"connectorIds\":[],\"side\":\"TOP\"},\"type\":\"ConnectorPlacement.EquallySpacedRectSide\",\"uuid\":\"0ff74274-cc13-4bc9-ab97-befa0144ddb0\"},{\"content\":{\"connectorIds\":[],\"side\":\"BOTTOM\"},\"type\":\"ConnectorPlacement.EquallySpacedRectSide\",\"uuid\":\"b4539d99-d74c-48ec-aeba-e1211e6ae847\"}]},\"type\":\"ConnectorPlacement.EquallySpacedConnector\",\"uuid\":\"32a64cae-dc0e-47e5-be72-f6041fa7e3a1\"}],\"packageUris\":[\"http://schema.mathworks.com/mf0/Connector/R2020b\"],\"version\":\"1.0\"}"
  Charge Socket : Subsystem
      settings: PortSchema="{\"entries\":[{\"content\":{\"headerSize\":26,\"margin\":15,\"minimumSpacing\":25,\"sides\":[{\"content\":{\"connectorIds\":[\"Out1\"]},\"type\":\"ConnectorPlacement.EquallySpacedRectSide\",\"uuid\":\"e97e1fd1-9f1b-43cc-bf15-a23fe97b9f57\"},{\"content\":{\"connectorIds\":[],\"side\":\"RIGHT\"},\"type\":\"ConnectorPlacement.EquallySpacedRectSide\",\"uuid\":\"b384b9c5-fcee-4054-b020-18cc4d409726\"},{\"content\":{\"connectorIds\":[],\"side\":\"TOP\"},\"type\":\"ConnectorPlacement.EquallySpacedRectSide\",\"uuid\":\"0ff74274-cc13-4bc9-ab97-befa0144ddb0\"}]},\"type\":\"ConnectorPlacement.EquallySpacedConnector\",\"uuid\":\"32a64cae-dc0e-47e5-be72-f6041fa7e3a1\"}],\"packageUris\":[\"http://schema.mathworks.com/mf0/Connector/R2020b\"],\"version\":\"1.0\"}"
  Drone Body : Subsystem
      settings: PortSchema="{\"entries\":[{\"content\":{\"headerSize\":26,\"margin\":15,\"minimumSpacing\":25,\"sides\":[{\"content\":{\"connectorIds\":[\"In4\",\"In5\",\"In6\",\"In7\",\"In9\",\"In10\",\"In11\",\"In12\",\"In13\"]},\"type\":\"ConnectorPlacement.EquallySpacedRectSide\",\"uuid\":\"e97e1fd1-9f1b-43cc-bf15-a23fe97b9f57\"},{\"content\":{\"connectorIds\":[\"Out1\",\"Out2\",\"Out3\",\"Out4\",\"Out5\",\"Out6\",\"Out7\"],\"side\":\"RIGHT\"},\"type\":\"ConnectorPlacement.EquallySpacedRectSide\",\"uuid\":\"b384b9c5-fcee-4054-b020-18cc4d409726\"},{\"content\":{\"connectorIds\":[\"In8\"],\"side\":\"TOP\"},\"type\":\"ConnectorPlacement.EquallySpacedRectSide\",\"uuid\":\"0ff74274-cc13-4bc9-ab97-befa0144ddb0\"},{\"content\":{\"connectorIds\":[\"In1\",\"In2\",\"In3\"],\"side\":\"BOTTOM\"},\"type\":\"ConnectorPlacement.EquallySpacedRectSide\",\"uuid\":\"7ce7253b-acc0-4f10-9339-933eaf6a63d7\"}]},\"type\":\"ConnectorPlacement.EquallySpacedConnector\",\"uuid\":\"32a64cae-dc0e-47e5-be72-f6041fa7e3a1\"}],\"packageUris\":[\"http://schema.mathworks.com/mf0/Connector/R2020b\"],\"version\":\"1.0\"}"
  Environment Perturbations : Subsystem
      settings: PortSchema="{\"entries\":[{\"content\":{\"headerSize\":26,\"margin\":15,\"minimumSpacing\":25,\"sides\":[{\"content\":{\"connectorIds\":[\"In1\"]},\"type\":\"ConnectorPlacement.EquallySpacedRectSide\",\"uuid\":\"e97e1fd1-9f1b-43cc-bf15-a23fe97b9f57\"},{\"content\":{\"connectorIds\":[\"Out1\",\"Out2\",\"Out3\"],\"side\":\"RIGHT\"},\"type\":\"ConnectorPlacement.EquallySpacedRectSide\",\"uuid\":\"b384b9c5-fcee-4054-b020-18cc4d409726\"},{\"content\":{\"connectorIds\":[],\"side\":\"TOP\"},\"type\":\"ConnectorPlacement.EquallySpacedRectSide\",\"uuid\":\"0ff74274-cc13-4bc9-ab97-befa0144ddb0\"}]},\"type\":\"ConnectorPlacement.EquallySpacedConnector\",\"uuid\":\"32a64cae-dc0e-47e5-be72-f6041fa7e3a1\"}],\"packageUris\":[\"http://schema.mathworks.com/mf0/Connector/R2020b\"],\"version\":\"1.0\"}"
  Flow Deck : Subsystem
      settings: PortSchema="{\"entries\":[{\"content\":{\"headerSize\":26,\"margin\":15,\"minimumSpacing\":25,\"sides\":[{\"content\":{\"connectorIds\":[]},\"type\":\"ConnectorPlacement.EquallySpacedRectSide\",\"uuid\":\"e97e1fd1-9f1b-43cc-bf15-a23fe97b9f57\"},{\"content\":{\"connectorIds\":[\"In1\",\"In2\"],\"side\":\"RIGHT\"},\"type\":\"ConnectorPlacement.EquallySpacedRectSide\",\"uuid\":\"b384b9c5-fcee-4054-b020-18cc4d409726\"},{\"content\":{\"connectorIds\":[],\"side\":\"TOP\"},\"type\":\"ConnectorPlacement.EquallySpacedRectSide\",\"uuid\":\"0ff74274-cc13-4bc9-ab97-befa0144ddb0\"},{\"content\":{\"connectorIds\":[\"Out1\",\"Out2\",\"Out3\"],\"side\":\"BOTTOM\"},\"type\":\"ConnectorPlacement.EquallySpacedRectSide\",\"uuid\":\"ab92106b-82a7-4521-8e33-681688d695ab\"}]},\"type\":\"ConnectorPlacement.EquallySpacedConnector\",\"uuid\":\"32a64cae-dc0e-47e5-be72-f6041fa7e3a1\"}],\"packageUris\":[\"http://schema.mathworks.com/mf0/Connector/R2020b\"],\"version\":\"1.0\"}"
  LED Ring Deck : Subsystem
      settings: PortSchema="{\"entries\":[{\"content\":{\"headerSize\":26,\"margin\":15,\"minimumSpacing\":25,\"sides\":[{\"content\":{\"connectorIds\":[\"In3\"]},\"type\":\"ConnectorPlacement.EquallySpacedRectSide\",\"uuid\":\"e97e1fd1-9f1b-43cc-bf15-a23fe97b9f57\"},{\"content\":{\"connectorIds\":[],\"side\":\"RIGHT\"},\"type\":\"ConnectorPlacement.EquallySpacedRectSide\",\"uuid\":\"b384b9c5-fcee-4054-b020-18cc4d409726\"},{\"content\":{\"connectorIds\":[],\"side\":\"TOP\"},\"type\":\"ConnectorPlacement.EquallySpacedRectSide\",\"uuid\":\"0ff74274-cc13-4bc9-ab97-befa0144ddb0\"},{\"content\":{\"connectorIds\":[\"In1\",\"In2\"],\"side\":\"BOTTOM\"},\"type\":\"ConnectorPlacement.EquallySpacedRectSide\",\"uuid\":\"87d33254-4794-497d-a279-1d76ceaafdba\"}]},\"type\":\"ConnectorPlacement.EquallySpacedConnector\",\"uuid\":\"32a64cae-dc0e-47e5-be72-f6041fa7e3a1\"}],\"packageUris\":[\"http://schema.mathworks.com/mf0/Connector/R2020b\"],\"version\":\"1.0\"}"
  Motor 1 : Subsystem
      settings: PortSchema="{\"entries\":[{\"content\":{\"headerSize\":26,\"margin\":15,\"minimumSpacing\":25,\"sides\":[{\"content\":{\"connectorIds\":[\"In2\",\"In3\"]},\"type\":\"ConnectorPlacement.EquallySpacedRectSide\",\"uuid\":\"e97e1fd1-9f1b-43cc-bf15-a23fe97b9f57\"},{\"content\":{\"connectorIds\":[\"In1\",\"Out1\"],\"side\":\"RIGHT\"},\"type\":\"ConnectorPlacement.EquallySpacedRectSide\",\"uuid\":\"b384b9c5-fcee-4054-b020-18cc4d409726\"},{\"content\":{\"connectorIds\":[],\"side\":\"TOP\"},\"type\":\"ConnectorPlacement.EquallySpacedRectSide\",\"uuid\":\"0ff74274-cc13-4bc9-ab97-befa0144ddb0\"}]},\"type\":\"ConnectorPlacement.EquallySpacedConnector\",\"uuid\":\"32a64cae-dc0e-47e5-be72-f6041fa7e3a1\"}],\"packageUris\":[\"http://schema.mathworks.com/mf0/Connector/R2020b\"],\"version\":\"1.0\"}"
  Motor 2 : Subsystem
      settings: PortSchema="{\"entries\":[{\"content\":{\"headerSize\":26,\"margin\":15,\"minimumSpacing\":25,\"sides\":[{\"content\":{\"connectorIds\":[\"In2\",\"In3\"]},\"type\":\"ConnectorPlacement.EquallySpacedRectSide\",\"uuid\":\"e97e1fd1-9f1b-43cc-bf15-a23fe97b9f57\"},{\"content\":{\"connectorIds\":[\"In1\",\"Out1\"],\"side\":\"RIGHT\"},\"type\":\"ConnectorPlacement.EquallySpacedRectSide\",\"uuid\":\"b384b9c5-fcee-4054-b020-18cc4d409726\"},{\"content\":{\"connectorIds\":[],\"side\":\"TOP\"},\"type\":\"ConnectorPlacement.EquallySpacedRectSide\",\"uuid\":\"0ff74274-cc13-4bc9-ab97-befa0144ddb0\"}]},\"type\":\"ConnectorPlacement.EquallySpacedConnector\",\"uuid\":\"32a64cae-dc0e-47e5-be72-f6041fa7e3a1\"}],\"packageUris\":[\"http://schema.mathworks.com/mf0/Connector/R2020b\"],\"version\":\"1.0\"}"
  Motor 3 : Subsystem
      settings: PortSchema="{\"entries\":[{\"content\":{\"headerSize\":26,\"margin\":15,\"minimumSpacing\":25,\"sides\":[{\"content\":{\"connectorIds\":[\"In2\",\"In3\"]},\"type\":\"ConnectorPlacement.EquallySpacedRectSide\",\"uuid\":\"e97e1fd1-9f1b-43cc-bf15-a23fe97b9f57\"},{\"content\":{\"connectorIds\":[\"In1\",\"Out1\"],\"side\":\"RIGHT\"},\"type\":\"ConnectorPlacement.EquallySpacedRectSide\",\"uuid\":\"b384b9c5-fcee-4054-b020-18cc4d409726\"},{\"content\":{\"connectorIds\":[],\"side\":\"TOP\"},\"type\":\"ConnectorPlacement.EquallySpacedRectSide\",\"uuid\":\"0ff74274-cc13-4bc9-ab97-befa0144ddb0\"}]},\"type\":\"ConnectorPlacement.EquallySpacedConnector\",\"uuid\":\"32a64cae-dc0e-47e5-be72-f6041fa7e3a1\"}],\"packageUris\":[\"http://schema.mathworks.com/mf0/Connector/R2020b\"],\"version\":\"1.0\"}"
  Motor 4 : Subsystem
      settings: PortSchema="{\"entries\":[{\"content\":{\"headerSize\":26,\"margin\":15,\"minimumSpacing\":25,\"sides\":[{\"content\":{\"connectorIds\":[\"In2\",\"In3\"]},\"type\":\"ConnectorPlacement.EquallySpacedRectSide\",\"uuid\":\"e97e1fd1-9f1b-43cc-bf15-a23fe97b9f57\"},{\"content\":{\"connectorIds\":[\"In1\",\"Out1\"],\"side\":\"RIGHT\"},\"type\":\"ConnectorPlacement.EquallySpacedRectSide\",\"uuid\":\"b384b9c5-fcee-4054-b020-18cc4d409726\"},{\"content\":{\"connectorIds\":[],\"side\":\"TOP\"},\"type\":\"ConnectorPlacement.EquallySpacedRectSide\",\"uuid\":\"0ff74274-cc13-4bc9-ab97-befa0144ddb0\"}]},\"type\":\"ConnectorPlacement.EquallySpacedConnector\",\"uuid\":\"32a64cae-dc0e-47e5-be72-f6041fa7e3a1\"}],\"packageUris\":[\"http://schema.mathworks.com/mf0/Connector/R2020b\"],\"version\":\"1.0\"}"
  Motor Arm 1 : Subsystem
      settings: PortSchema="{\"entries\":[{\"content\":{\"headerSize\":26,\"margin\":15,\"minimumSpacing\":25,\"sides\":[{\"content\":{\"connectorIds\":[\"In1\"]},\"type\":\"ConnectorPlacement.EquallySpacedRectSide\",\"uuid\":\"e97e1fd1-9f1b-43cc-bf15-a23fe97b9f57\"},{\"content\":{\"connectorIds\":[\"Out1\"],\"side\":\"RIGHT\"},\"type\":\"ConnectorPlacement.EquallySpacedRectSide\",\"uuid\":\"b384b9c5-fcee-4054-b020-18cc4d409726\"},{\"content\":{\"connectorIds\":[],\"side\":\"TOP\"},\"type\":\"ConnectorPlacement.EquallySpacedRectSide\",\"uuid\":\"0ff74274-cc13-4bc9-ab97-befa0144ddb0\"}]},\"type\":\"ConnectorPlacement.EquallySpacedConnector\",\"uuid\":\"32a64cae-dc0e-47e5-be72-f6041fa7e3a1\"}],\"packageUris\":[\"http://schema.mathworks.com/mf0/Connector/R2020b\"],\"version\":\"1.0\"}"
  Motor Arm 2 : Subsystem
      settings: PortSchema="{\"entries\":[{\"content\":{\"headerSize\":26,\"margin\":15,\"minimumSpacing\":25,\"sides\":[{\"content\":{\"connectorIds\":[\"In1\"]},\"type\":\"ConnectorPlacement.EquallySpacedRectSide\",\"uuid\":\"e97e1fd1-9f1b-43cc-bf15-a23fe97b9f57\"},{\"content\":{\"connectorIds\":[\"Out1\"],\"side\":\"RIGHT\"},\"type\":\"ConnectorPlacement.EquallySpacedRectSide\",\"uuid\":\"b384b9c5-fcee-4054-b020-18cc4d409726\"},{\"content\":{\"connectorIds\":[],\"side\":\"TOP\"},\"type\":\"ConnectorPlacement.EquallySpacedRectSide\",\"uuid\":\"0ff74274-cc13-4bc9-ab97-befa0144ddb0\"}]},\"type\":\"ConnectorPlacement.EquallySpacedConnector\",\"uuid\":\"32a64cae-dc0e-47e5-be72-f6041fa7e3a1\"}],\"packageUris\":[\"http://schema.mathworks.com/mf0/Connector/R2020b\"],\"version\":\"1.0\"}"
  Motor Arm 3 : Subsystem
      settings: PortSchema="{\"entries\":[{\"content\":{\"headerSize\":26,\"margin\":15,\"minimumSpacing\":25,\"sides\":[{\"content\":{\"connectorIds\":[\"In1\"]},\"type\":\"ConnectorPlacement.EquallySpacedRectSide\",\"uuid\":\"e97e1fd1-9f1b-43cc-bf15-a23fe97b9f57\"},{\"content\":{\"connectorIds\":[\"Out1\"],\"side\":\"RIGHT\"},\"type\":\"ConnectorPlacement.EquallySpacedRectSide\",\"uuid\":\"b384b9c5-fcee-4054-b020-18cc4d409726\"},{\"content\":{\"connectorIds\":[],\"side\":\"TOP\"},\"type\":\"ConnectorPlacement.EquallySpacedRectSide\",\"uuid\":\"0ff74274-cc13-4bc9-ab97-befa0144ddb0\"}]},\"type\":\"ConnectorPlacement.EquallySpacedConnector\",\"uuid\":\"32a64cae-dc0e-47e5-be72-f6041fa7e3a1\"}],\"packageUris\":[\"http://schema.mathworks.com/mf0/Connector/R2020b\"],\"version\":\"1.0\"}"
  Motor Arm 4 : Subsystem
      settings: PortSchema="{\"entries\":[{\"content\":{\"headerSize\":26,\"margin\":15,\"minimumSpacing\":25,\"sides\":[{\"content\":{\"connectorIds\":[\"In1\"]},\"type\":\"ConnectorPlacement.EquallySpacedRectSide\",\"uuid\":\"e97e1fd1-9f1b-43cc-bf15-a23fe97b9f57\"},{\"content\":{\"connectorIds\":[\"Out1\"],\"side\":\"RIGHT\"},\"type\":\"ConnectorPlacement.EquallySpacedRectSide\",\"uuid\":\"b384b9c5-fcee-4054-b020-18cc4d409726\"},{\"content\":{\"connectorIds\":[],\"side\":\"TOP\"},\"type\":\"ConnectorPlacement.EquallySpacedRectSide\",\"uuid\":\"0ff74274-cc13-4bc9-ab97-befa0144ddb0\"}]},\"type\":\"ConnectorPlacement.EquallySpacedConnector\",\"uuid\":\"32a64cae-dc0e-47e5-be72-f6041fa7e3a1\"}],\"packageUris\":[\"http://schema.mathworks.com/mf0/Connector/R2020b\"],\"version\":\"1.0\"}"
  Power Supply Board : Subsystem
      settings: PortSchema="{\"entries\":[{\"content\":{\"headerSize\":26,\"margin\":15,\"minimumSpacing\":25,\"sides\":[{\"content\":{\"connectorIds\":[\"In2\"]},\"type\":\"ConnectorPlacement.EquallySpacedRectSide\",\"uuid\":\"e97e1fd1-9f1b-43cc-bf15-a23fe97b9f57\"},{\"content\":{\"connectorIds\":[\"In1\"],\"side\":\"RIGHT\"},\"type\":\"ConnectorPlacement.EquallySpacedRectSide\",\"uuid\":\"b384b9c5-fcee-4054-b020-18cc4d409726\"},{\"content\":{\"connectorIds\":[\"Out1\"],\"side\":\"TOP\"},\"type\":\"ConnectorPlacement.EquallySpacedRectSide\",\"uuid\":\"0ff74274-cc13-4bc9-ab97-befa0144ddb0\"},{\"content\":{\"connectorIds\":[],\"side\":\"BOTTOM\"},\"type\":\"ConnectorPlacement.EquallySpacedRectSide\",\"uuid\":\"809e6a72-aa6e-4b5a-9bf6-9a2695eaa733\"}]},\"type\":\"ConnectorPlacement.EquallySpacedConnector\",\"uuid\":\"32a64cae-dc0e-47e5-be72-f6041fa7e3a1\"}],\"packageUris\":[\"http://schema.mathworks.com/mf0/Connector/R2020b\"],\"version\":\"1.0\"}"
  Bus Element Out1 : Outport  PortName=Telemetry
  Bus Element Out2 : Outport  Port=2  PortName=FPVVideo
  wires:
  Motor 4/1(rotate) -> CW Helix 2/1(rotate)
  Motor Arm 4/1(hold) -> Motor 4/3(hold)
  Motor Arm 3/1(hold) -> Motor 3/3(hold)
  Motor 3/1(rotate) -> CCW Helix 2/1(rotate)
  Motor 1/1(rotate) -> CCW Helix 1/1(rotate)
  Drone Body/2(hold0) -> Motor Arm 2/1(hold0), Motor Arm 4/1(hold0), Motor Arm 3/1(hold0), Motor Arm 1/1(hold0)
  Motor Arm 1/1(hold) -> Motor 1/3(hold)
  Battery/1(Power) -> Power Supply Board/2(Bat_Power)
  Motor Arm 2/1(hold) -> Motor 2/3(hold)
  Motor 2/1(rotate) -> CW Helix 1/1(rotate)
  Drone Body/1(MalePins) -> AI-deck/2(MalePins), LED Ring Deck/1(MalePins), Flow Deck/1(MalePins), Battery Holder Deck/1(MalePins)
  Battery Holder Deck/1(hold) -> Battery/1(hold)
  Charge Socket/1(Power) -> Power Supply Board/1(Power)
  Power Supply Board/1(5 V) -> Motor 2/1(Power), Motor 4/1(Power), Motor 3/1(Power), Motor 1/1(Power), Drone Body/8(Power), LED Ring Deck/2(Power), Flow Deck/2(Power), AI-deck/3(Power)
  Bus Element In3/1 -> Environment Perturbations/1(environment)
  Drone Body/4(Motor1_PWM) -> Motor 1/2(Motor1_PWM)
  Drone Body/5(Motor2_PWM) -> Motor 2/2(Motor2_PWM)
  Drone Body/6(Motor3_PWM) -> Motor 3/2(Motor3_PWM)
  Drone Body/7(Motor4_PWM) -> Motor 4/2(Motor4_PWM)
  AI-deck/1(VideoBus) -> Bus Element Out2/1
  Bus Element In8/1 -> AI-deck/1(obs)
  Bus Element In9/1 -> LED Ring Deck/3(LED_cmds)
  Bus Element In2/1 -> Drone Body/7(GCS)
  Flow Deck/1(dx) -> Drone Body/6(dx)
  Flow Deck/2(dy) -> Drone Body/5(dy)
  Flow Deck/3(z) -> Drone Body/4(z)
  Environment Perturbations/1(F_x_in) -> Drone Body/1(F_x_in)
  Environment Perturbations/2(F_y_in) -> Drone Body/2(F_y_in)
  Environment Perturbations/3(F_z_in) -> Drone Body/3(F_z_in)
  Drone Body/3(Telemetry) -> Bus Element Out1/1
  Bus Element In4/1 -> Drone Body/9(z_mob)
  Bus Element In5/1 -> Drone Body/10(pitch_mob)
  Bus Element In6/1 -> Drone Body/11(roll_mob)
  Bus Element In7/1 -> Drone Body/12(yaw_mob)
  Bus Element In1/1 -> Drone Body/13(TelemetryRadio)

== system Hell_ix_System_Architecture/Hell-ix/CrazyRadio PA ==
  Bus Element In1 : Inport  PortName=Telemetry_USB
  Bus Element In2 : Inport  Port=2  PortName=GCSCmds
  Bus Element Out1 : Outport  PortName=TelemetryRadio
  Bus Element Out2 : Outport  Port=2  PortName=GCS

== system Hell_ix_System_Architecture/Hell-ix/Ground Control Station ==
  Bus Element In5 : Inport  PortName=config
  Bus Element In1 : Inport  Port=2  PortName=exec_prog
  Bus Element In4 : Inport  Port=3  PortName=FPVVideo
  Bus Element In3 : Inport  Port=4  PortName=Telemetry
  Commands : Subsystem
      settings: PortSchema="{\"entries\":[{\"content\":{\"headerSize\":26,\"margin\":15,\"minimumSpacing\":25,\"sides\":[{\"content\":{\"connectorIds\":[\"In1\",\"In2\",\"In3\",\"In4\",\"In5\"]},\"type\":\"ConnectorPlacement.EquallySpacedRectSide\",\"uuid\":\"b8d7d09c-e9ae-43de-8d46-f99ec2351e24\"},{\"content\":{\"connectorIds\":[\"Out1\",\"Out2\"],\"side\":\"RIGHT\"},\"type\":\"ConnectorPlacement.EquallySpacedRectSide\",\"uuid\":\"4693648e-b0a2-4db8-a983-4bee2f51d894\"},{\"content\":{\"connectorIds\":[],\"side\":\"TOP\"},\"type\":\"ConnectorPlacement.EquallySpacedRectSide\",\"uuid\":\"9f0e5fe3-4fa7-4597-a4df-94b2d5032736\"}]},\"type\":\"ConnectorPlacement.EquallySpacedConnector\",\"uuid\":\"297bf07a-4341-4423-8aed-0af6edbe7857\"}],\"packageUris\":[\"http://schema.mathworks.com/mf0/Connector/R2020b\"],\"version\":\"1.0\"}"
  Program Selection : Subsystem  Variant=on  VariantControlMode=label  LabelModeActiveChoice=true
      settings: PortSchema="{\"entries\":[{\"content\":{\"headerSize\":38,\"margin\":15,\"minimumSpacing\":25,\"sides\":[{\"content\":{\"connectorIds\":[\"In1\",\"In2\",\"In3\"]},\"type\":\"ConnectorPlacement.EquallySpacedRectSide\",\"uuid\":\"61491797-d554-4a74-923e-4bee7d1a8f93\"},{\"content\":{\"connectorIds\":[\"Out1\",\"Out2\",\"Out3\",\"Out4\",\"Out5\"],\"side\":\"RIGHT\"},\"type\":\"ConnectorPlacement.EquallySpacedRectSide\",\"uuid\":\"68e3b5ad-c508-4145-a439-f07408910c2d\"},{\"content\":{\"connectorIds\":[],\"side\":\"TOP\"},\"type\":\"ConnectorPlacement.EquallySpacedRectSide\",\"uuid\":\"f52cb127-a246-45d5-a620-fd9d5ecf46f3\"}]},\"type\":\"ConnectorPlacement.EquallySpacedConnector\",\"uuid\":\"13f104e8-deb7-48c1-a5c8-cc1a7de63fd1\"}],\"packageUris\":[\"http://schema.mathworks.com/mf0/Connector/R2020b\"],\"version\":\"1.0\"}"
  Bus Element Out1 : Outport  PortName=Telemetry_USB
  Bus Element Out2 : Outport  Port=2  PortName=GCSCmds
  wires:
  Bus Element In5/1 -> Program Selection/1(config)
  Bus Element In1/1 -> Program Selection/2(exec_prog)
  Bus Element In4/1 -> Program Selection/3(FPVVideo)
  Program Selection/1(pos_x_out) -> Commands/1(pos_x_out)
  Program Selection/2(pos_y_out) -> Commands/2(pos_y_out)
  Program Selection/3(pos_z_out) -> Commands/3(pos_z_out)
  Program Selection/4(yaw_out) -> Commands/4(yaw_out)
  Commands/1(Telemetry_USB) -> Bus Element Out1/1
  Commands/2(GCSCmds) -> Bus Element Out2/1
  Program Selection/5(LED_conf) -> Commands/5(LED_conf)

== system Hell_ix_System_Architecture/Hell-ix/cfclient Mobile Phone ==
  Bus Element Out1 : Outport  PortName=z_mob
  Bus Element Out2 : Outport  Port=2  PortName=pitch_mob
  Bus Element Out4 : Outport  Port=3  PortName=roll_mob
  Bus Element Out3 : Outport  Port=4  PortName=yaw_mob
